simulink model "call_model"  (R2022a)
settings: Solver=ode113  StartTime=0.0  StopTime=7000  RelTol=1e-5
values from neighbouring files (symbols this model uses):
  k = 2.0    (= 2)    [process.m]
  kd = kdata(i,2)    [process.m]
  ki = kdata(i,1)    [process.m]
  kp = kdata(i,3)    [process.m]
  target = data(1,2)    [process.m]
  Tm = 0.6    [process.m]
settings Model: Creator=Xu  LastModifiedBy=Xu
settings SolverCC: ZeroCrossAlgorithm=Adaptive

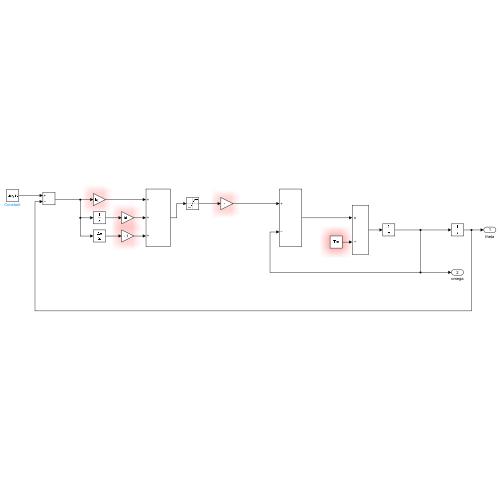
[thumbnail: Simulink's stored preview of the top-level diagram]
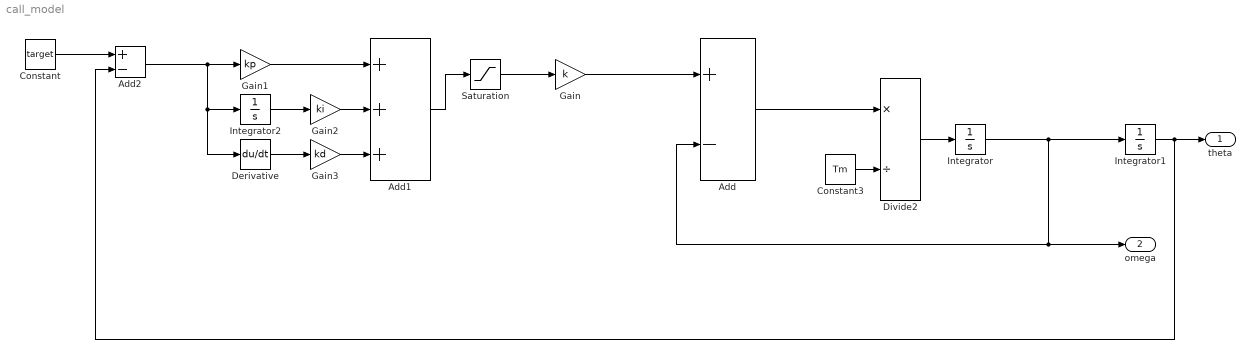
== system call_model ==
  Add : Sum  Inputs=+-
  Add1 : Sum  Inputs=+++
  Add2 : Sum  Inputs=+-
  Constant : Constant  Value=target
  Constant3 : Constant  Value=Tm
  Derivative : Derivative
  Divide2 : Product  Inputs=*/
  Gain : Gain  Gain=k
  Gain1 : Gain  Gain=kp
  Gain2 : Gain  Gain=ki
  Gain3 : Gain  Gain=kd
  Integrator : Integrator
  Integrator1 : Integrator
  Integrator2 : Integrator
  Saturation : Saturate  UpperLimit=7  LowerLimit=-7
  theta : Outport
  omega : Outport  Port=2
  wires:
  Gain/1 -> Add/1
  Add/1 -> Divide2/1
  Constant3/1 -> Divide2/2
  Divide2/1 -> Integrator/1
  Integrator/1 -> omega/1, Add/2, Integrator1/1
  Integrator1/1 -> theta/1, Add2/2
  Saturation/1 -> Gain/1
  Add1/1 -> Saturation/1
  Add2/1 -> Derivative/1, Integrator2/1, Gain1/1
  Constant/1 -> Add2/1
  Gain1/1 -> Add1/1
  Integrator2/1 -> Gain2/1
  Derivative/1 -> Gain3/1
  Gain2/1 -> Add1/2
  Gain3/1 -> Add1/3
